simulink model "S_S_annotated"  (R2022b)
settings: Solver=VariableStepAuto  StartTime=0.0  StopTime=10e-3  RelTol=1e-3
libraries: spsVoltageMeasurementLib x6, spsCurrentMeasurementLib x4, spsMosfetLib x4, spsSeriesRLCBranchLib x4, eeRmsMeasurement x3, spsDCVoltageSourceLib x1, spsMutualInductanceLib x1, spsUniversalBridgeLib x1, spspowerguiLib x1
settings Model: Creator=赵健  LastModifiedBy=Dongjunfeng
settings SolverCC: AlgebraicLoopSolver=TrustRegion
settings DebuggingCC: UnconnectedInputMsg=warning  UnconnectedOutputMsg=warning  UnconnectedLineMsg=warning  SFMachineParentedDataDiag=warning
settings ModelReferenceCC: EnableRefExpFcnMdlSchedulingChecks=on
settings RTWCC: DLArmComputeVersion=19.05

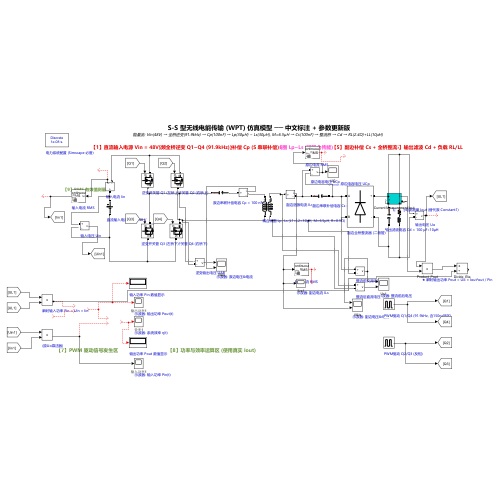
[thumbnail: Simulink's stored preview of the top-level diagram]
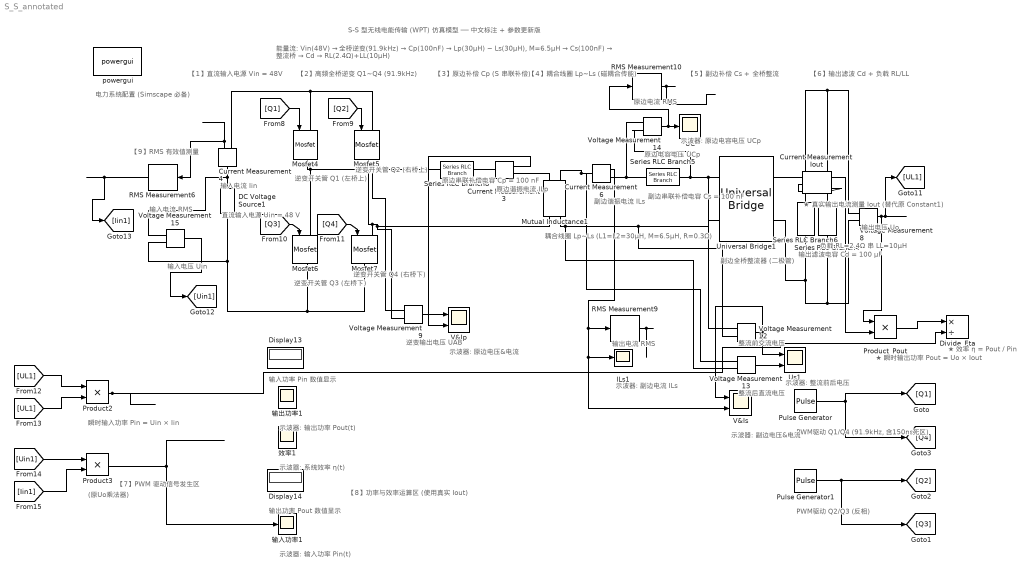
== system S_S_annotated ==
  note: 直流输入电源 Uin = 48 V
  note: 逆变开关管 Q1 (左桥上)
  note: 逆变开关管 Q2 (右桥上)
  note: 逆变开关管 Q3 (左桥下)
  note: 逆变开关管 Q4 (右桥下)
  note: PWM驱动 Q1/Q4 (91.9kHz, 含150ns死区)
  note: PWM驱动 Q2/Q3 (反相)
  note: 原边串联补偿电容 Cp = 100 nF
  note: 耦合线圈 Lp~Ls (L1=L2=30µH, M=6.5µH, R=0.3Ω)
  note: 副边串联补偿电容 Cs = 100 nF
  note: 副边全桥整流器 (二极管)
  note: 输出滤波电容 Cd = 100 µF
  note: 负载 RL=2.4Ω 串 LL=10µH
  note: ★ 真实输出电流测量 Iout (替代原 Constant1)
  note: 输入电流 Iin
  note: 原边谐振电流 ILp
  note: 副边谐振电流 ILs
  note: 输入电压 Uin
  note: 逆变输出电压 UAB
  note: 原边电容电压 UCp
  note: 整流前交流电压
  note: 整流后直流电压
  note: 输出电压 Uo
  note: 输入电流 RMS
  note: 原边电流 RMS
  note: 输出电流 RMS
  note: 瞬时输入功率 Pin = Uin × Iin
  note: (原Uo乘法器)
  note: ★ 瞬时输出功率 Pout = Uo × Iout
  note: ★ 效率 η = Pout / Pin
  note: 输入功率 Pin 数值显示
  note: 输出功率 Pout 数值显示
  note: 示波器: 副边电流 ILs
  note: 示波器: 原边电容电压 UCp
  note: 示波器: 整流前后电压
  note: 示波器: 原边电压&电流
  note: 示波器: 副边电压&电流
  note: 示波器: 系统效率 η(t)
  note: 示波器: 输入功率 Pin(t)
  note: 示波器: 输出功率 Pout(t)
  note: 电力系统配置 (Simscape 必备)
  note: 【1】直流输入电源 Vin = 48V
  note: 【2】高频全桥逆变 Q1~Q4 (91.9kHz)
  note: 【3】原边补偿 Cp (S 串联补偿)
  note: 【4】耦合线圈 Lp~Ls (磁耦合传能)
  note: 【5】副边补偿 Cs + 全桥整流
  note: 【6】输出滤波 Cd + 负载 RL/LL
  note: 【7】PWM 驱动信号发生区
  note: 【8】功率与效率运算区 (使用真实 Iout)
  note: 【9】RMS 有效值测量
  note: S-S 型无线电能传输 (WPT) 仿真模型 ── 中文标注 + 参数更新版
  note: 能量流: Vin(48V) → 全桥逆变(91.9kHz) → Cp(100nF) → Lp(30µH) ~ Ls(30µH), M=6.5µH → Cs(100nF) → 整流桥 → Cd → RL(2.4Ω)+LL(10µH)
  Current Measurement Iout : spsCurrentMeasurementLib/Current Measurement  Description=★ 真实输出电流测量 Iout (替代原 Constant1)  PhasorSimulation=off  OutputType=Complex  PSBequivalent=0
  Current Measurement3 : spsCurrentMeasurementLib/Current Measurement  Description=原边谐振电流 ILp  PhasorSimulation=off  OutputType=Complex  PSBequivalent=0
  Current Measurement4 : spsCurrentMeasurementLib/Current Measurement  Description=输入电流 Iin  PhasorSimulation=off  OutputType=Complex  PSBequivalent=0
  Current Measurement6 : spsCurrentMeasurementLib/Current Measurement  Description=副边谐振电流 ILs  PhasorSimulation=off  OutputType=Complex  PSBequivalent=0
  DC Voltage Source1 : spsDCVoltageSourceLib/DC Voltage Source  Description=直流输入电源 Uin = 48 V  Amplitude=48  Measurements=None
  Display13 : Display
      settings: Description=输入功率 Pin 数值显示
  Display14 : Display
      settings: Description=输出功率 Pout 数值显示
  Divide_Eta : Product  Description=★ 效率 η = Pout / Pin  Inputs=*/
  ILs1 : Scope
      settings: Description=示波器: 副边电流 ILs
  Mosfet4 : spsMosfetLib/Mosfet  Description=逆变开关管 Q1 (左桥上)  Ron=0.044  Lon=0  Rd=0.01  Vfd=0  IC=0  Rs=1e5  Cs=inf  Measurements=off
  Mosfet5 : spsMosfetLib/Mosfet  Description=逆变开关管 Q2 (右桥上)  Ron=0.044  Lon=0  Rd=0.01  Vfd=0  IC=0  Rs=1e5  Cs=inf  Measurements=off
  Mosfet6 : spsMosfetLib/Mosfet  Description=逆变开关管 Q3 (左桥下)  Ron=0.044  Lon=0  Rd=0.01  Vfd=0  IC=0  Rs=1e5  Cs=inf  Measurements=off
  Mosfet7 : spsMosfetLib/Mosfet  Description=逆变开关管 Q4 (右桥下)  Ron=0.044  Lon=0  Rd=0.01  Vfd=0  IC=0  Rs=1e5  Cs=inf  Measurements=off
  Mutual Inductance1 : spsMutualInductanceLib/Mutual Inductance  Description=耦合线圈 Lp~Ls (L1=L2=30µH, M=6.5µH, R=0.3Ω)  LConnTagsString=a|b  RConnTagsString=A|B  TypeOfMutual=Two or three windings with equal mutual terms  NumberOfWindings=2  SelfImpedance1=[0.3 30e-6]  SelfImpedance2=[0.3 30e-6]  ThreeWindings=off  SelfImpedance3=[ 1.1 1.1e-03]  MutualImpedance=[0 6.5e-6]  InductanceMatrix="[1.0 0.9  0.9 ;  0.9 1.0  0.9;  0.9 0.9 1.0 ] * 1e-3"  ResistanceMatrix="[1.0 0.9  0.9 ;  0.9 1.0  0.9;  0.9 0.9 1.0 ]"  Measurements=None
  Product2 : Product  Description=瞬时输入功率 Pin = Uin × Iin
  Product3 : Product  Description=(原Uo乘法器)
  Product_Pout : Product  Description=★ 瞬时输出功率 Pout = Uo × Iout  Inputs=**
  Pulse Generator : DiscretePulseGenerator  Description=PWM驱动 Q1/Q4 (91.9kHz, 含150ns死区)  PulseType=Time based  Period=1/91900  PulseWidth=48.6215
  Pulse Generator1 : DiscretePulseGenerator  Description=PWM驱动 Q2/Q3 (反相)  PulseType=Time based  Period=1/91900  PulseWidth=48.6215  PhaseDelay=1/91900/2
  RMS Measurement10 : eeRmsMeasurement/RMS Measurement  Description=原边电流 RMS  LabelModeActiveChoice=Total  F=100000  SpecifyHarmonics=off  K=[0 1 2]  Ts=0
  RMS Measurement6 : eeRmsMeasurement/RMS Measurement  Description=输入电流 RMS  LabelModeActiveChoice=Total  F=100000  SpecifyHarmonics=off  K=[0 1 2]  Ts=0
  RMS Measurement9 : eeRmsMeasurement/RMS Measurement  Description=输出电流 RMS  LabelModeActiveChoice=Total  F=100000  SpecifyHarmonics=off  K=[0 1 2]  Ts=0
  Series RLC Branch4 : spsSeriesRLCBranchLib/Series RLC Branch  Description=负载 RL=2.4Ω 串 LL=10µH  LConnTagsString=__new0  RConnTagsString=__new0  BranchType=RL  Resistance=2.4  Inductance=10e-6  SetiL0=off  InitialCurrent=0  Capacitance=1e-6  Setx0=off  InitialVoltage=0  Measurements=None
  Series RLC Branch5 : spsSeriesRLCBranchLib/Series RLC Branch  Description=副边串联补偿电容 Cs = 100 nF  LConnTagsString=__new0  RConnTagsString=__new0  BranchType=C  Resistance=0.023  Inductance=1e-3  SetiL0=off  InitialCurrent=0  Capacitance=100e-9  Setx0=off  InitialVoltage=0  Measurements=None
  Series RLC Branch6 : spsSeriesRLCBranchLib/Series RLC Branch  Description=输出滤波电容 Cd = 100 µF  LConnTagsString=__new0  RConnTagsString=__new0  BranchType=C  Resistance=0.05  Inductance=1e-3  SetiL0=off  InitialCurrent=0  Capacitance=100e-6  Setx0=off  InitialVoltage=0  Measurements=None
  Series RLC Branch8 : spsSeriesRLCBranchLib/Series RLC Branch  Description=原边串联补偿电容 Cp = 100 nF  LConnTagsString=__new0  RConnTagsString=__new0  BranchType=C  Resistance=0.023  Inductance=1e-3  SetiL0=off  InitialCurrent=0  Capacitance=100e-9  Setx0=off  InitialVoltage=0  Measurements=None
  UC : Scope
      settings: Description=示波器: 原边电容电压 UCp
  Universal Bridge1 : spsUniversalBridgeLib/Universal Bridge  Description=副边全桥整流器 (二极管)  Arms=2  SnubberResistance=1e5  SnubberCapacitance=inf  Device=Diodes  Ron=1e-3  Lon=0  ForwardVoltages="[  0  0  ]"  ForwardVoltage=0  GTOparameters=[ 10e-6 , 20e-6 ]  IGBTparameters=[ 1e-6 , 2e-6 ]  Measurements=None  Measurements_2=None  converterType=Rectifier
  Us1 : Scope  NumInputPorts=2
      settings: Description=示波器: 整流前后电压
  V&Ip : Scope  NumInputPorts=2
      settings: Description=示波器: 原边电压&电流
  V&Is : Scope  NumInputPorts=2
      settings: Description=示波器: 副边电压&电流
  Voltage Measurement12 : spsVoltageMeasurementLib/Voltage Measurement  Description=整流前交流电压  PhasorSimulation=off  OutputType=Complex  PSBequivalent=0
  Voltage Measurement13 : spsVoltageMeasurementLib/Voltage Measurement  Description=整流后直流电压  PhasorSimulation=off  OutputType=Complex  PSBequivalent=0
  Voltage Measurement14 : spsVoltageMeasurementLib/Voltage Measurement  Description=原边电容电压 UCp  PhasorSimulation=off  OutputType=Complex  PSBequivalent=0
  Voltage Measurement15 : spsVoltageMeasurementLib/Voltage Measurement  Description=输入电压 Uin  PhasorSimulation=off  OutputType=Complex  PSBequivalent=0
  Voltage Measurement8 : spsVoltageMeasurementLib/Voltage Measurement  Description=输出电压 Uo  PhasorSimulation=off  OutputType=Complex  PSBequivalent=0
  Voltage Measurement9 : spsVoltageMeasurementLib/Voltage Measurement  Description=逆变输出电压 UAB  PhasorSimulation=off  OutputType=Complex  PSBequivalent=0
  powergui : spspowerguiLib/powergui  Description=电力系统配置 (Simscape 必备)  Priority=1  SimulationMode=Discrete  SampleTime=1e-8  frequency=60  Iterations=50  frequencyindice=0  Pbase=100e6  ErrMax=1e-4  UnitsV=kV  UnitsW=MW  buscounter=0  FunctionMessages=off  echomessages=off  EnableUseOfTLC=off  CurrentSourceSwitches=off  DisableSnubberDevices=off  DisableRonSwitches=off  DisableVfSwitches=off  DisplayEquations=off  AutomaticDiscreteSolvers=off  SolverType=Tustin/Backward Euler (TBE)  Interpol=off  ExternalGateDelay=off  methode=off  Ts=10  x0status=blocks  SPID=off  SwTol=0  HookPort=off  NonlinearTolerance=0  nMaxIteration=15  ContinueOnMaxIteration=off  RestoreLinks=warning  ResistiveCurrentMeasurement=off  Frange=[0:2:500]  Ylog=off  Xlog=on  ShowGrid=off  save=off  variable=ZData  structure=0  ZoomFFT=off  StartTime=0.0  cycles=1  DisplayStyle=1  fundamental=60  FreqAxis=off  MaxFrequency=1000  frequencyindicesteady=1  RmsSteady=1  display=off
  效率1 : Scope
      settings: Description=示波器: 系统效率 η(t)
  输入功率1 : Scope
      settings: Description=示波器: 输入功率 Pin(t)
  输出功率1 : Scope
      settings: Description=示波器: 输出功率 Pout(t)
  wires:
  ? -> Display13/1, 输出功率1/1
  Voltage Measurement15/1 -> [Uin1]
  [UL1] -> Product2/1
  [Q4] -> Mosfet7/1
  RMS Measurement9/1 -> ?
  [Iin1] -> Product3/2
  Current Measurement4/1 -> RMS Measurement6/1
  Voltage Measurement14/1 -> RMS Measurement10/1, UC/1
  [Q1] -> Mosfet4/1
  Current Measurement6/1 -> V&Is/2, ILs1/1, RMS Measurement9/1
  Voltage Measurement8/1 -> [UL1], Product_Pout/1
  Voltage Measurement9/1 -> V&Ip/1
  Voltage Measurement12/1 -> V&Is/1, Us1/1
  Pulse Generator1/1 -> [Q3], [Q2]
  Pulse Generator/1 -> [Q1], [Q4]
  [Q2] -> Mosfet5/1
  Current Measurement3/1 -> V&Ip/2
  [Uin1] -> Product3/1
  RMS Measurement6/1 -> [Iin1]
  Product3/1 -> 输入功率1/1
  ? -> Display14/1, 效率1/1
  RMS Measurement10/1 -> ?
  Voltage Measurement13/1 -> Us1/2
  [Q3] -> Mosfet6/1
  Product2/1 -> Divide_Eta/2
  ? -> ?
  [UL1] -> Product2/2
  Current Measurement Iout/1 -> Product_Pout/2
  Product_Pout/1 -> Divide_Eta/1
  connections:
  Current Measurement6/LConn1 -- Voltage Measurement13/LConn1 -- Mutual Inductance1/LConn2
  Mosfet4/RConn1 -- Mosfet6/LConn1 -- Series RLC Branch8/LConn1 -- Voltage Measurement9/LConn1
  DC Voltage Source1/LConn1 -- Mosfet7/RConn1 -- Mosfet6/RConn1 -- Voltage Measurement15/LConn2
  Voltage Measurement9/LConn2 -- Mutual Inductance1/RConn1 -- Mosfet5/RConn1 -- Mosfet7/LConn1
  Voltage Measurement12/LConn2 -- Voltage Measurement13/LConn2 -- Mutual Inductance1/RConn2 -- Universal Bridge1/LConn2
  Voltage Measurement12/LConn1 -- Series RLC Branch5/RConn1 -- Voltage Measurement14/LConn2 -- Universal Bridge1/LConn1
  Voltage Measurement14/LConn1 -- Current Measurement6/RConn1 -- Series RLC Branch5/LConn1
  Current Measurement4/RConn1 -- Mosfet5/LConn1 -- Mosfet4/LConn1
  Voltage Measurement15/LConn1 -- DC Voltage Source1/RConn1 -- Current Measurement4/LConn1
  Series RLC Branch6/RConn1 -- Voltage Measurement8/LConn2 -- Series RLC Branch4/RConn1 -- Universal Bridge1/RConn2
  Universal Bridge1/RConn1 -- Voltage Measurement8/LConn1 -- Series RLC Branch4/LConn1 -- Current Measurement Iout/RConn1 -- Series RLC Branch6/LConn1 -- Current Measurement Iout/LConn1
  Current Measurement3/RConn1 -- Mutual Inductance1/LConn1
  Series RLC Branch8/RConn1 -- Current Measurement3/LConn1
